simulink model "decController"  (R2015b)
settings: Solver=FixedStepAuto  StartTime=0.0  StopTime=inf  RelTol=1e-3
libraries: robotlib x24, simulink x6
settings Model: Creator=rasrack  LastModifiedBy=rasrack
settings OptimizationCC: OptimizeModelRefInitCode=on  MaxStackSize=64
settings HardwareCC: ProdBitPerPointer=32  ProdLargestAtomicFloat=None  ProdIntDivRoundTo=Undefined  ProdEndianess=Unspecified  ProdWordSize=32  ProdHWDeviceType=Generic->Unspecified (assume 32-bit Generic)
settings RTWCC: SystemTargetFile=ert.tlc  TemplateMakefile=ert_default_tmf  Description=Embedded Coder  Toolchain=Catkin  TargetLang=C++
settings CodeAppCC: IgnoreCustomStorageClasses=off

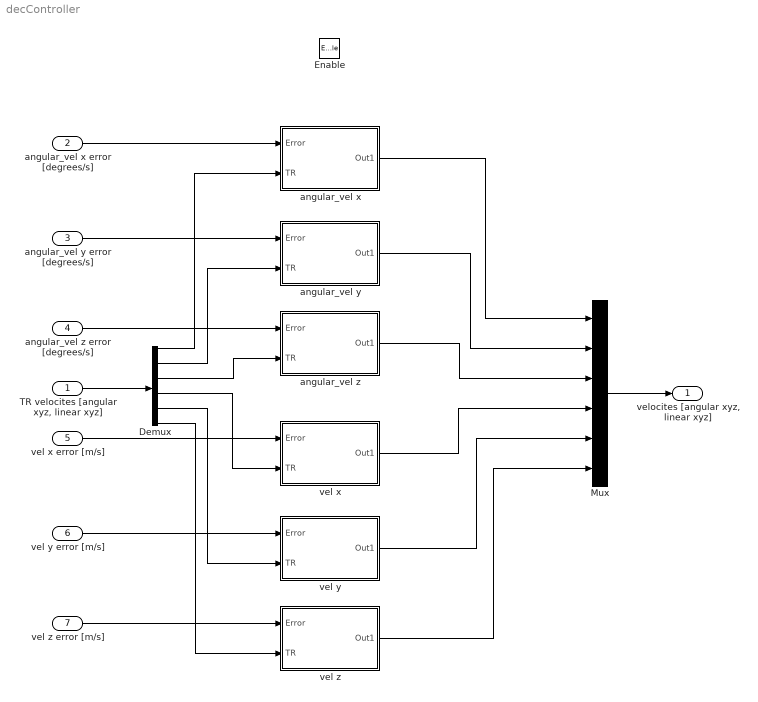
== system decController ==
  "TR velocites [angular xyz, linear xyz]  " : Inport
  "angular_vel x error [degrees/s] " : Inport  Port=2
  angular_vel y error [degrees/s] : Inport  Port=3
  angular_vel z error [degrees/s] : Inport  Port=4
  "vel x error [m/s] " : Inport  Port=5
  "vel y error [m/s] " : Inport  Port=6
  "vel z error [m/s] " : Inport  Port=7
  Enable : EnablePort
  Demux : Demux  Outputs=6
  Mux : Mux  Inputs=6
  angular_vel x : Subsystem
  angular_vel y : Subsystem
  angular_vel z : Subsystem
  vel x : Subsystem
  vel y : Subsystem
  vel z : Subsystem
  "velocites [angular xyz, linear xyz]" : Outport
  wires:
  "angular_vel x error [degrees/s] "/1 -> angular_vel x/1(Error)
  angular_vel y error [degrees/s]/1 -> angular_vel y/1(Error)
  angular_vel z error [degrees/s]/1 -> angular_vel z/1(Error)
  "vel x error [m/s] "/1 -> vel x/1(Error)
  "vel y error [m/s] "/1 -> vel y/1(Error)
  "vel z error [m/s] "/1 -> vel z/1(Error)
  vel z/1(Out1) -> Mux/6
  angular_vel x/1(Out1) -> Mux/1
  angular_vel y/1(Out1) -> Mux/2
  angular_vel z/1(Out1) -> Mux/3
  vel x/1(Out1) -> Mux/4
  vel y/1(Out1) -> Mux/5
  Mux/1 -> "velocites [angular xyz, linear xyz]"/1
  "TR velocites [angular xyz, linear xyz]  "/1 -> Demux/1
  Demux/1 -> angular_vel x/2(TR)
  Demux/2 -> angular_vel y/2(TR)
  Demux/3 -> angular_vel z/2(TR)
  Demux/4 -> vel x/2(TR)
  Demux/5 -> vel y/2(TR)
  Demux/6 -> vel z/2(TR)

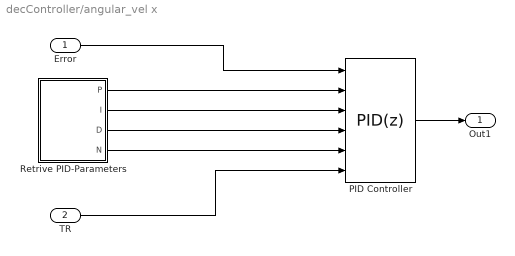
== system decController/angular_vel x ==
  Error : Inport
  TR : Inport  Port=2
  PID Controller : simulink/Continuous/PID Controller  Controller=PID  TimeDomain=Discrete-time  SampleTime=-1  IntegratorMethod=Forward Euler  FilterMethod=Forward Euler  Form=Parallel  UseFilter=on  ControllerParametersSource=external  P=1  I=1  D=0  N=100  InitialConditionSource=internal  InitialConditionForIntegrator=0  InitialConditionForFilter=0  ExternalReset=none  LimitOutput=on  UpperSaturationLimit=1  LowerSaturationLimit=-1  LinearizeAsGain=on  AntiWindupMode=clamping  Kb=1  TrackingMode=on  Kt=1  SaturateOnIntegerOverflow=on  PParamMin=[]  PParamMax=[]  IParamMin=[]  IParamMax=[]  DParamMin=[]  DParamMax=[]  NParamMin=[]  NParamMax=[]  KbParamMin=[]  KbParamMax=[]  KtParamMin=[]  KtParamMax=[]  POutMin=[]  POutMax=[]  IOutMin=[]  IOutMax=[]  DOutMin=[]  DOutMax=[]  NOutMin=[]  NOutMax=[]  KbOutMin=[]  KbOutMax=[]  KtOutMin=[]  KtOutMax=[]  IntegratorOutMin=[]  IntegratorOutMax=[]  FilterOutMin=[]  FilterOutMax=[]  SumOutMin=[]  SumOutMax=[]  SumI1OutMin=[]  SumI1OutMax=[]  SumI2OutMin=[]  SumI2OutMax=[]  SumI3OutMin=[]  SumI3OutMax=[]  SumDOutMin=[]  SumDOutMax=[]  SaturationOutMin=[]  SaturationOutMax=[]  SaturationOutDataTypeStr=double  IntegratorContinuousStateAttributes=''  IntegratorStateMustResolveToSignalObject=off  IntegratorRTWStateStorageClass=Auto  FilterContinuousStateAttributes=''  FilterStateMustResolveToSignalObject=off  FilterRTWStateStorageClass=Auto  DifferentiatorICPrevScaledInput=0  DifferentiatorOutMin=[]  DifferentiatorOutMax=[]
  Retrive PID-Parameters : Subsystem
  Out1 : Outport
  wires:
  Retrive PID-Parameters/3(D) -> PID Controller/4
  Retrive PID-Parameters/2(I) -> PID Controller/3
  Retrive PID-Parameters/4(N) -> PID Controller/5
  Retrive PID-Parameters/1(P) -> PID Controller/2
  TR/1 -> PID Controller/6
  Error/1 -> PID Controller/1
  PID Controller/1 -> Out1/1

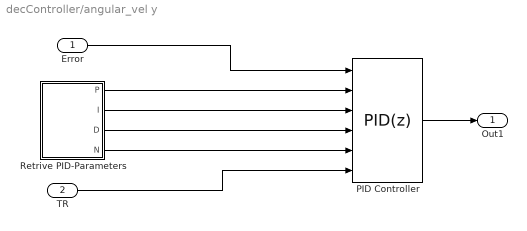
== system decController/angular_vel y ==
  Error : Inport
  TR : Inport  Port=2
  PID Controller : simulink/Continuous/PID Controller  Controller=PID  TimeDomain=Discrete-time  SampleTime=-1  IntegratorMethod=Forward Euler  FilterMethod=Forward Euler  Form=Parallel  UseFilter=on  ControllerParametersSource=external  P=1  I=1  D=0  N=100  InitialConditionSource=internal  InitialConditionForIntegrator=0  InitialConditionForFilter=0  ExternalReset=none  LimitOutput=on  UpperSaturationLimit=1  LowerSaturationLimit=-1  LinearizeAsGain=on  AntiWindupMode=clamping  Kb=1  TrackingMode=on  Kt=1  SaturateOnIntegerOverflow=on  PParamMin=[]  PParamMax=[]  IParamMin=[]  IParamMax=[]  DParamMin=[]  DParamMax=[]  NParamMin=[]  NParamMax=[]  KbParamMin=[]  KbParamMax=[]  KtParamMin=[]  KtParamMax=[]  POutMin=[]  POutMax=[]  IOutMin=[]  IOutMax=[]  DOutMin=[]  DOutMax=[]  NOutMin=[]  NOutMax=[]  KbOutMin=[]  KbOutMax=[]  KtOutMin=[]  KtOutMax=[]  IntegratorOutMin=[]  IntegratorOutMax=[]  FilterOutMin=[]  FilterOutMax=[]  SumOutMin=[]  SumOutMax=[]  SumI1OutMin=[]  SumI1OutMax=[]  SumI2OutMin=[]  SumI2OutMax=[]  SumI3OutMin=[]  SumI3OutMax=[]  SumDOutMin=[]  SumDOutMax=[]  SaturationOutMin=[]  SaturationOutMax=[]  IntegratorContinuousStateAttributes=''  IntegratorStateMustResolveToSignalObject=off  IntegratorRTWStateStorageClass=Auto  FilterContinuousStateAttributes=''  FilterStateMustResolveToSignalObject=off  FilterRTWStateStorageClass=Auto  DifferentiatorICPrevScaledInput=0  DifferentiatorOutMin=[]  DifferentiatorOutMax=[]
  Retrive PID-Parameters : Subsystem
  Out1 : Outport
  wires:
  Retrive PID-Parameters/3(D) -> PID Controller/4
  Retrive PID-Parameters/2(I) -> PID Controller/3
  Retrive PID-Parameters/4(N) -> PID Controller/5
  Retrive PID-Parameters/1(P) -> PID Controller/2
  TR/1 -> PID Controller/6
  Error/1 -> PID Controller/1
  PID Controller/1 -> Out1/1

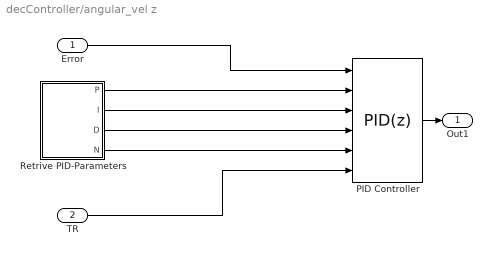
== system decController/angular_vel z ==
  Error : Inport
  TR : Inport  Port=2
  PID Controller : simulink/Continuous/PID Controller  Controller=PID  TimeDomain=Discrete-time  SampleTime=-1  IntegratorMethod=Forward Euler  FilterMethod=Forward Euler  Form=Parallel  UseFilter=on  ControllerParametersSource=external  P=1  I=1  D=0  N=100  InitialConditionSource=internal  InitialConditionForIntegrator=0  InitialConditionForFilter=0  ExternalReset=none  LimitOutput=on  UpperSaturationLimit=1  LowerSaturationLimit=-1  LinearizeAsGain=on  AntiWindupMode=clamping  Kb=1  TrackingMode=on  Kt=1  SaturateOnIntegerOverflow=on  PParamMin=[]  PParamMax=[]  IParamMin=[]  IParamMax=[]  DParamMin=[]  DParamMax=[]  NParamMin=[]  NParamMax=[]  KbParamMin=[]  KbParamMax=[]  KtParamMin=[]  KtParamMax=[]  POutMin=[]  POutMax=[]  IOutMin=[]  IOutMax=[]  DOutMin=[]  DOutMax=[]  NOutMin=[]  NOutMax=[]  KbOutMin=[]  KbOutMax=[]  KtOutMin=[]  KtOutMax=[]  IntegratorOutMin=[]  IntegratorOutMax=[]  FilterOutMin=[]  FilterOutMax=[]  SumOutMin=[]  SumOutMax=[]  SumI1OutMin=[]  SumI1OutMax=[]  SumI2OutMin=[]  SumI2OutMax=[]  SumI3OutMin=[]  SumI3OutMax=[]  SumDOutMin=[]  SumDOutMax=[]  SaturationOutMin=[]  SaturationOutMax=[]  IntegratorContinuousStateAttributes=''  IntegratorStateMustResolveToSignalObject=off  IntegratorRTWStateStorageClass=Auto  FilterContinuousStateAttributes=''  FilterStateMustResolveToSignalObject=off  FilterRTWStateStorageClass=Auto  DifferentiatorICPrevScaledInput=0  DifferentiatorOutMin=[]  DifferentiatorOutMax=[]
  Retrive PID-Parameters : Subsystem
  Out1 : Outport
  wires:
  Retrive PID-Parameters/3(D) -> PID Controller/4
  Retrive PID-Parameters/2(I) -> PID Controller/3
  Retrive PID-Parameters/4(N) -> PID Controller/5
  Retrive PID-Parameters/1(P) -> PID Controller/2
  TR/1 -> PID Controller/6
  Error/1 -> PID Controller/1
  PID Controller/1 -> Out1/1

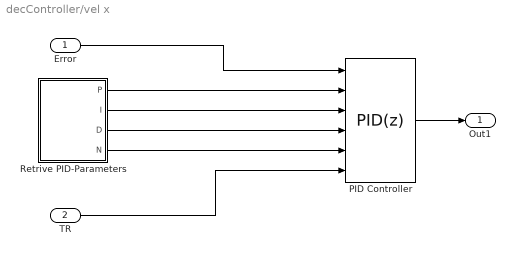
== system decController/vel x ==
  Error : Inport
  TR : Inport  Port=2
  PID Controller : simulink/Continuous/PID Controller  Controller=PID  TimeDomain=Discrete-time  SampleTime=-1  IntegratorMethod=Forward Euler  FilterMethod=Forward Euler  Form=Parallel  UseFilter=on  ControllerParametersSource=external  P=1  I=1  D=0  N=100  InitialConditionSource=internal  InitialConditionForIntegrator=0  InitialConditionForFilter=0  ExternalReset=none  LimitOutput=on  UpperSaturationLimit=1  LowerSaturationLimit=-1  LinearizeAsGain=on  AntiWindupMode=clamping  Kb=1  TrackingMode=on  Kt=1  SaturateOnIntegerOverflow=on  PParamMin=[]  PParamMax=[]  IParamMin=[]  IParamMax=[]  DParamMin=[]  DParamMax=[]  NParamMin=[]  NParamMax=[]  KbParamMin=[]  KbParamMax=[]  KtParamMin=[]  KtParamMax=[]  POutMin=[]  POutMax=[]  IOutMin=[]  IOutMax=[]  DOutMin=[]  DOutMax=[]  NOutMin=[]  NOutMax=[]  KbOutMin=[]  KbOutMax=[]  KtOutMin=[]  KtOutMax=[]  IntegratorOutMin=[]  IntegratorOutMax=[]  FilterOutMin=[]  FilterOutMax=[]  SumOutMin=[]  SumOutMax=[]  SumI1OutMin=[]  SumI1OutMax=[]  SumI2OutMin=[]  SumI2OutMax=[]  SumI3OutMin=[]  SumI3OutMax=[]  SumDOutMin=[]  SumDOutMax=[]  SaturationOutMin=[]  SaturationOutMax=[]  IntegratorContinuousStateAttributes=''  IntegratorStateMustResolveToSignalObject=off  IntegratorRTWStateStorageClass=Auto  FilterContinuousStateAttributes=''  FilterStateMustResolveToSignalObject=off  FilterRTWStateStorageClass=Auto  DifferentiatorICPrevScaledInput=0  DifferentiatorOutMin=[]  DifferentiatorOutMax=[]
  Retrive PID-Parameters : Subsystem
  Out1 : Outport
  wires:
  Retrive PID-Parameters/3(D) -> PID Controller/4
  Retrive PID-Parameters/2(I) -> PID Controller/3
  Retrive PID-Parameters/4(N) -> PID Controller/5
  Retrive PID-Parameters/1(P) -> PID Controller/2
  TR/1 -> PID Controller/6
  Error/1 -> PID Controller/1
  PID Controller/1 -> Out1/1

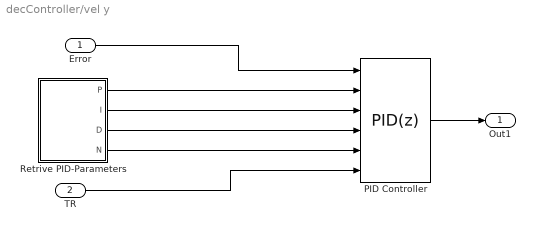
== system decController/vel y ==
  Error : Inport
  TR : Inport  Port=2
  PID Controller : simulink/Continuous/PID Controller  Controller=PID  TimeDomain=Discrete-time  SampleTime=-1  IntegratorMethod=Forward Euler  FilterMethod=Forward Euler  Form=Parallel  UseFilter=on  ControllerParametersSource=external  P=1  I=1  D=0  N=100  InitialConditionSource=internal  InitialConditionForIntegrator=0  InitialConditionForFilter=0  ExternalReset=none  LimitOutput=on  UpperSaturationLimit=1  LowerSaturationLimit=-1  LinearizeAsGain=on  AntiWindupMode=clamping  Kb=1  TrackingMode=on  Kt=1  SaturateOnIntegerOverflow=on  PParamMin=[]  PParamMax=[]  IParamMin=[]  IParamMax=[]  DParamMin=[]  DParamMax=[]  NParamMin=[]  NParamMax=[]  KbParamMin=[]  KbParamMax=[]  KtParamMin=[]  KtParamMax=[]  POutMin=[]  POutMax=[]  IOutMin=[]  IOutMax=[]  DOutMin=[]  DOutMax=[]  NOutMin=[]  NOutMax=[]  KbOutMin=[]  KbOutMax=[]  KtOutMin=[]  KtOutMax=[]  IntegratorOutMin=[]  IntegratorOutMax=[]  FilterOutMin=[]  FilterOutMax=[]  SumOutMin=[]  SumOutMax=[]  SumI1OutMin=[]  SumI1OutMax=[]  SumI2OutMin=[]  SumI2OutMax=[]  SumI3OutMin=[]  SumI3OutMax=[]  SumDOutMin=[]  SumDOutMax=[]  SaturationOutMin=[]  SaturationOutMax=[]  IntegratorContinuousStateAttributes=''  IntegratorStateMustResolveToSignalObject=off  IntegratorRTWStateStorageClass=Auto  FilterContinuousStateAttributes=''  FilterStateMustResolveToSignalObject=off  FilterRTWStateStorageClass=Auto  DifferentiatorICPrevScaledInput=0  DifferentiatorOutMin=[]  DifferentiatorOutMax=[]
  Retrive PID-Parameters : Subsystem
  Out1 : Outport
  wires:
  Retrive PID-Parameters/3(D) -> PID Controller/4
  Retrive PID-Parameters/2(I) -> PID Controller/3
  Retrive PID-Parameters/4(N) -> PID Controller/5
  Retrive PID-Parameters/1(P) -> PID Controller/2
  TR/1 -> PID Controller/6
  Error/1 -> PID Controller/1
  PID Controller/1 -> Out1/1

== system decController/vel z ==
  Error : Inport
  TR : Inport  Port=2
  PID Controller : simulink/Continuous/PID Controller  Controller=PID  TimeDomain=Discrete-time  SampleTime=-1  IntegratorMethod=Forward Euler  FilterMethod=Forward Euler  Form=Parallel  UseFilter=on  ControllerParametersSource=external  P=1  I=1  D=0  N=100  InitialConditionSource=internal  InitialConditionForIntegrator=0  InitialConditionForFilter=0  ExternalReset=none  LimitOutput=on  UpperSaturationLimit=1  LowerSaturationLimit=-1  LinearizeAsGain=on  AntiWindupMode=clamping  Kb=1  TrackingMode=on  Kt=1  SaturateOnIntegerOverflow=on  PParamMin=[]  PParamMax=[]  IParamMin=[]  IParamMax=[]  DParamMin=[]  DParamMax=[]  NParamMin=[]  NParamMax=[]  KbParamMin=[]  KbParamMax=[]  KtParamMin=[]  KtParamMax=[]  POutMin=[]  POutMax=[]  IOutMin=[]  IOutMax=[]  DOutMin=[]  DOutMax=[]  NOutMin=[]  NOutMax=[]  KbOutMin=[]  KbOutMax=[]  KtOutMin=[]  KtOutMax=[]  IntegratorOutMin=[]  IntegratorOutMax=[]  FilterOutMin=[]  FilterOutMax=[]  SumOutMin=[]  SumOutMax=[]  SumI1OutMin=[]  SumI1OutMax=[]  SumI2OutMin=[]  SumI2OutMax=[]  SumI3OutMin=[]  SumI3OutMax=[]  SumDOutMin=[]  SumDOutMax=[]  SaturationOutMin=[]  SaturationOutMax=[]  IntegratorContinuousStateAttributes=''  IntegratorStateMustResolveToSignalObject=off  IntegratorRTWStateStorageClass=Auto  FilterContinuousStateAttributes=''  FilterStateMustResolveToSignalObject=off  FilterRTWStateStorageClass=Auto  DifferentiatorICPrevScaledInput=0  DifferentiatorOutMin=[]  DifferentiatorOutMax=[]
  Retrive PID-Parameters : Subsystem
  Out1 : Outport
  wires:
  Retrive PID-Parameters/3(D) -> PID Controller/4
  Retrive PID-Parameters/2(I) -> PID Controller/3
  Retrive PID-Parameters/4(N) -> PID Controller/5
  Retrive PID-Parameters/1(P) -> PID Controller/2
  TR/1 -> PID Controller/6
  Error/1 -> PID Controller/1
  PID Controller/1 -> Out1/1

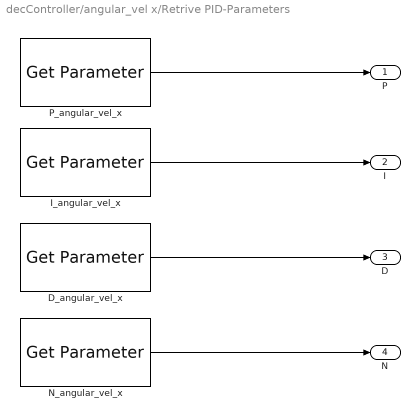
== system decController/angular_vel x/Retrive PID-Parameters ==
  D_angular_vel_x : robotlib/Get Parameter  SourceLibraryInfo=This block requires Robotics System Toolbox  ParameterSource=Select from ROS network  ParameterName=/matlab_controller/D_angular_vel_x  ParameterType=double  ParameterInitialValue=0  SampleTime=-1  ShowErrorCodeOutput=off  ModelName=decController  BlockId=ParamGet_decController_13
  I_angular_vel_x : robotlib/Get Parameter  SourceLibraryInfo=This block requires Robotics System Toolbox  ParameterSource=Select from ROS network  ParameterName=/matlab_controller/I_angular_vel_x  ParameterType=double  ParameterInitialValue=0  SampleTime=-1  ShowErrorCodeOutput=off  ModelName=decController  BlockId=ParamGet_decController_14
  "N_angular_vel_x " : robotlib/Get Parameter  SourceLibraryInfo=This block requires Robotics System Toolbox  ParameterSource=Specify your own  ParameterName=/matlab_controller/N_angular_vel_x  ParameterType=double  ParameterInitialValue=0  SampleTime=-1  ShowErrorCodeOutput=off  ModelName=decController  BlockId=ParamGet_decController_15
  P_angular_vel_x : robotlib/Get Parameter  SourceLibraryInfo=This block requires Robotics System Toolbox  ParameterSource=Select from ROS network  ParameterName=/matlab_controller/P_angular_vel_x  ParameterType=double  ParameterInitialValue=0  SampleTime=-1  ShowErrorCodeOutput=off  ModelName=decController  BlockId=ParamGet_decController_16
  P : Outport
  I : Outport  Port=2
  D : Outport  Port=3
  N : Outport  Port=4
  wires:
  "N_angular_vel_x "/1 -> N/1
  D_angular_vel_x/1 -> D/1
  I_angular_vel_x/1 -> I/1
  P_angular_vel_x/1 -> P/1

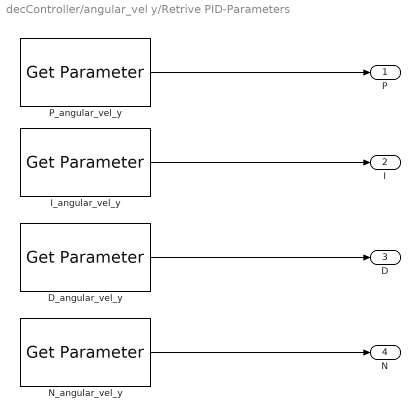
== system decController/angular_vel y/Retrive PID-Parameters ==
  D_angular_vel_y : robotlib/Get Parameter  SourceLibraryInfo=This block requires Robotics System Toolbox  ParameterSource=Specify your own  ParameterName=/matlab_controller/D_angular_vel_y  ParameterType=double  ParameterInitialValue=0  SampleTime=-1  ShowErrorCodeOutput=off  ModelName=decController  BlockId=ParamGet_decController_27
  I_angular_vel_y : robotlib/Get Parameter  SourceLibraryInfo=This block requires Robotics System Toolbox  ParameterSource=Specify your own  ParameterName=/matlab_controller/I_angular_vel_y  ParameterType=double  ParameterInitialValue=0  SampleTime=-1  ShowErrorCodeOutput=off  ModelName=decController  BlockId=ParamGet_decController_28
  "N_angular_vel_y " : robotlib/Get Parameter  SourceLibraryInfo=This block requires Robotics System Toolbox  ParameterSource=Specify your own  ParameterName=/matlab_controller/N_angular_vel_y  ParameterType=double  ParameterInitialValue=0  SampleTime=-1  ShowErrorCodeOutput=off  ModelName=decController  BlockId=ParamGet_decController_29
  P_angular_vel_y : robotlib/Get Parameter  SourceLibraryInfo=This block requires Robotics System Toolbox  ParameterSource=Specify your own  ParameterName=/matlab_controller/P_angular_vel_y  ParameterType=double  ParameterInitialValue=0  SampleTime=-1  ShowErrorCodeOutput=off  ModelName=decController  BlockId=ParamGet_decController_30
  P : Outport
  I : Outport  Port=2
  D : Outport  Port=3
  N : Outport  Port=4
  wires:
  "N_angular_vel_y "/1 -> N/1
  D_angular_vel_y/1 -> D/1
  I_angular_vel_y/1 -> I/1
  P_angular_vel_y/1 -> P/1

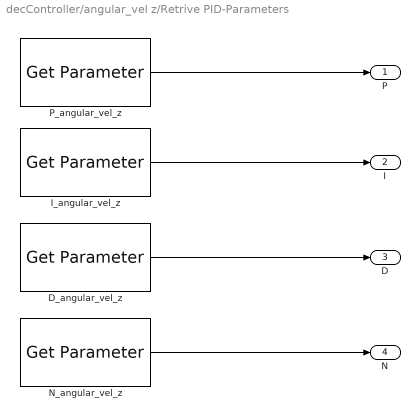
== system decController/angular_vel z/Retrive PID-Parameters ==
  D_angular_vel_z : robotlib/Get Parameter  SourceLibraryInfo=This block requires Robotics System Toolbox  ParameterSource=Specify your own  ParameterName=/matlab_controller/D_angular_vel_z  ParameterType=double  ParameterInitialValue=0  SampleTime=-1  ShowErrorCodeOutput=off  ModelName=decController  BlockId=ParamGet_decController_41
  I_angular_vel_z : robotlib/Get Parameter  SourceLibraryInfo=This block requires Robotics System Toolbox  ParameterSource=Specify your own  ParameterName=/matlab_controller/I_angular_vel_z  ParameterType=double  ParameterInitialValue=0  SampleTime=-1  ShowErrorCodeOutput=off  ModelName=decController  BlockId=ParamGet_decController_42
  "N_angular_vel_z " : robotlib/Get Parameter  SourceLibraryInfo=This block requires Robotics System Toolbox  ParameterSource=Specify your own  ParameterName=/matlab_controller/N_angular_vel_z  ParameterType=double  ParameterInitialValue=0  SampleTime=-1  ShowErrorCodeOutput=off  ModelName=decController  BlockId=ParamGet_decController_43
  P_angular_vel_z : robotlib/Get Parameter  SourceLibraryInfo=This block requires Robotics System Toolbox  ParameterSource=Specify your own  ParameterName=/matlab_controller/P_angular_vel_z  ParameterType=double  ParameterInitialValue=0  SampleTime=-1  ShowErrorCodeOutput=off  ModelName=decController  BlockId=ParamGet_decController_44
  P : Outport
  I : Outport  Port=2
  D : Outport  Port=3
  N : Outport  Port=4
  wires:
  "N_angular_vel_z "/1 -> N/1
  D_angular_vel_z/1 -> D/1
  I_angular_vel_z/1 -> I/1
  P_angular_vel_z/1 -> P/1

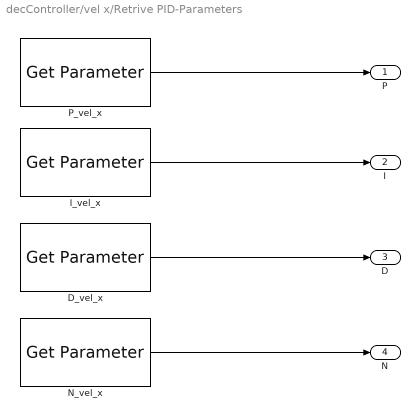
== system decController/vel x/Retrive PID-Parameters ==
  D_vel_x : robotlib/Get Parameter  SourceLibraryInfo=This block requires Robotics System Toolbox  ParameterSource=Specify your own  ParameterName=/matlab_controller/D_vel_x  ParameterType=double  ParameterInitialValue=0  SampleTime=-1  ShowErrorCodeOutput=off  ModelName=decController  BlockId=ParamGet_decController_55
  I_vel_x : robotlib/Get Parameter  SourceLibraryInfo=This block requires Robotics System Toolbox  ParameterSource=Specify your own  ParameterName=/matlab_controller/I_vel_x  ParameterType=double  ParameterInitialValue=0  SampleTime=-1  ShowErrorCodeOutput=off  ModelName=decController  BlockId=ParamGet_decController_56
  "N_vel_x " : robotlib/Get Parameter  SourceLibraryInfo=This block requires Robotics System Toolbox  ParameterSource=Specify your own  ParameterName=/matlab_controller/N_vel_x  ParameterType=double  ParameterInitialValue=0  SampleTime=-1  ShowErrorCodeOutput=off  ModelName=decController  BlockId=ParamGet_decController_57
  P_vel_x : robotlib/Get Parameter  SourceLibraryInfo=This block requires Robotics System Toolbox  ParameterSource=Specify your own  ParameterName=/matlab_controller/P_vel_x  ParameterType=double  ParameterInitialValue=0  SampleTime=-1  ShowErrorCodeOutput=off  ModelName=decController  BlockId=ParamGet_decController_58
  P : Outport
  I : Outport  Port=2
  D : Outport  Port=3
  N : Outport  Port=4
  wires:
  "N_vel_x "/1 -> N/1
  D_vel_x/1 -> D/1
  I_vel_x/1 -> I/1
  P_vel_x/1 -> P/1

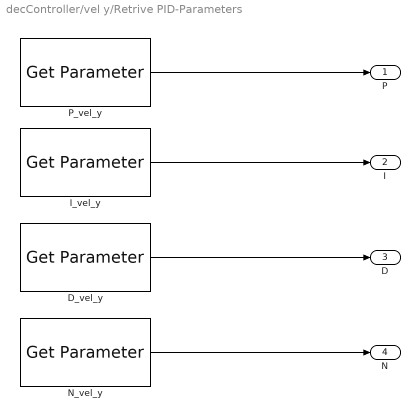
== system decController/vel y/Retrive PID-Parameters ==
  D_vel_y : robotlib/Get Parameter  SourceLibraryInfo=This block requires Robotics System Toolbox  ParameterSource=Specify your own  ParameterName=/matlab_controller/D_vel_y  ParameterType=double  ParameterInitialValue=0  SampleTime=-1  ShowErrorCodeOutput=off  ModelName=decController  BlockId=ParamGet_decController_69
  I_vel_y : robotlib/Get Parameter  SourceLibraryInfo=This block requires Robotics System Toolbox  ParameterSource=Specify your own  ParameterName=/matlab_controller/I_vel_y  ParameterType=double  ParameterInitialValue=0  SampleTime=-1  ShowErrorCodeOutput=off  ModelName=decController  BlockId=ParamGet_decController_70
  "N_vel_y " : robotlib/Get Parameter  SourceLibraryInfo=This block requires Robotics System Toolbox  ParameterSource=Specify your own  ParameterName=/matlab_controller/N_vel_y  ParameterType=double  ParameterInitialValue=0  SampleTime=-1  ShowErrorCodeOutput=off  ModelName=decController  BlockId=ParamGet_decController_71
  P_vel_y : robotlib/Get Parameter  SourceLibraryInfo=This block requires Robotics System Toolbox  ParameterSource=Specify your own  ParameterName=/matlab_controller/P_vel_y  ParameterType=double  ParameterInitialValue=0  SampleTime=-1  ShowErrorCodeOutput=off  ModelName=decController  BlockId=ParamGet_decController_72
  P : Outport
  I : Outport  Port=2
  D : Outport  Port=3
  N : Outport  Port=4
  wires:
  "N_vel_y "/1 -> N/1
  D_vel_y/1 -> D/1
  I_vel_y/1 -> I/1
  P_vel_y/1 -> P/1

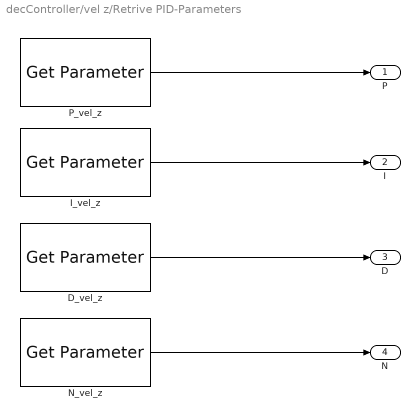
== system decController/vel z/Retrive PID-Parameters ==
  D_vel_z : robotlib/Get Parameter  SourceLibraryInfo=This block requires Robotics System Toolbox  ParameterSource=Specify your own  ParameterName=/matlab_controller/D_vel_z  ParameterType=double  ParameterInitialValue=0  SampleTime=-1  ShowErrorCodeOutput=off  ModelName=decController  BlockId=ParamGet_decController_83
  I_vel_z : robotlib/Get Parameter  SourceLibraryInfo=This block requires Robotics System Toolbox  ParameterSource=Specify your own  ParameterName=/matlab_controller/I_vel_z  ParameterType=double  ParameterInitialValue=0  SampleTime=-1  ShowErrorCodeOutput=off  ModelName=decController  BlockId=ParamGet_decController_84
  "N_vel_z " : robotlib/Get Parameter  SourceLibraryInfo=This block requires Robotics System Toolbox  ParameterSource=Specify your own  ParameterName=/matlab_controller/N_vel_z  ParameterType=double  ParameterInitialValue=0  SampleTime=-1  ShowErrorCodeOutput=off  ModelName=decController  BlockId=ParamGet_decController_85
  P_vel_z : robotlib/Get Parameter  SourceLibraryInfo=This block requires Robotics System Toolbox  ParameterSource=Specify your own  ParameterName=/matlab_controller/P_vel_z  ParameterType=double  ParameterInitialValue=0  SampleTime=-1  ShowErrorCodeOutput=off  ModelName=decController  BlockId=ParamGet_decController_86
  P : Outport
  I : Outport  Port=2
  D : Outport  Port=3
  N : Outport  Port=4
  wires:
  "N_vel_z "/1 -> N/1
  D_vel_z/1 -> D/1
  I_vel_z/1 -> I/1
  P_vel_z/1 -> P/1
